simulink model "modelo_motor_P4_2"  (R2021b)
settings: Solver=VariableStepAuto  StartTime=0.0  StopTime=Tend  RelTol=1e-3
values from neighbouring files (symbols this model uses):
  Kd = Kp*Td    (= 0.01)    [lanza_P4_2.m]
  Ki = Kp/Ti    (= 8.33333333333)    [lanza_P4_2.m]
  Kp = 5    [lanza_P4_2.m]
  Td = 0.002    [lanza_P4_2.m]
  Ti = 0.6    [lanza_P4_2.m]
  Tm = 0.01    [lanza_P4_1.m]    (also in lanza_P4_2.m)
undefined symbols (not defined in the file or in its folder): k_bc, V_sat
libraries: cstblocks x6, slpidlib x1, dspsrcs4 x1
settings Model: Creator=jvalls  LastModifiedBy=jgragia
settings SolverCC: AlgebraicLoopSolver=TrustRegion
settings DataIOCC: ReturnWorkspaceOutputs=off
settings DebuggingCC: SFMachineParentedDataDiag=warning  ArithmeticOperatorsInVariantConditions=warning
settings SFSimCC: SimUseLocalCustomCode=off  CustomCodeUndefinedFunction=UseInterfaceOnly
settings RTWCC: RTWUseLocalCustomCode=off

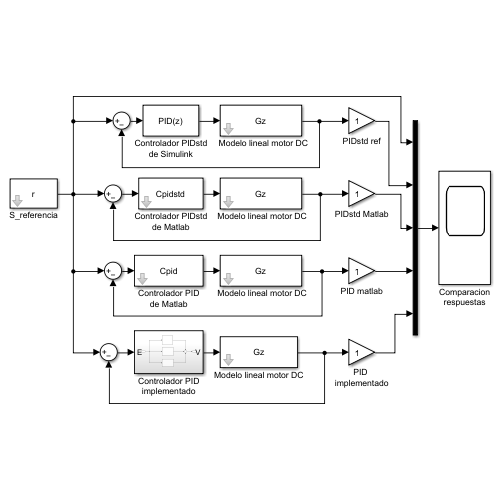
[thumbnail: Simulink's stored preview of the top-level diagram]
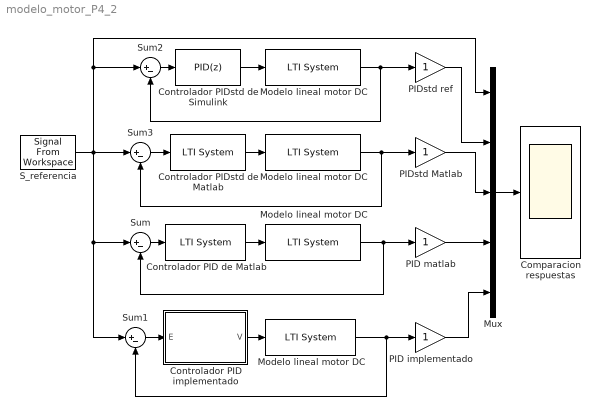
== system modelo_motor_P4_2 ==
  "       Modelo lineal motor DC      " : cstblocks/LTI System  sys=Gz  IC=[]
  "     Modelo lineal motor DC    " : cstblocks/LTI System  sys=Gz  IC=[]
  "    Modelo lineal motor DC  " : cstblocks/LTI System  sys=Gz  IC=[]
  "  Modelo lineal motor DC  " : cstblocks/LTI System  sys=Gz  IC=[]
  Comparacion respuestas : Scope
  Controlador PID de Matlab : cstblocks/LTI System  sys=Cpid  IC=[]
  Controlador PID implementado : Subsystem
  Controlador PIDstd de Matlab : cstblocks/LTI System  sys=Cpidstd  IC=[]
  Controlador PIDstd de Simulink : slpidlib/PID Controller  Controller=PID  Form=Ideal  TimeDomain=Discrete-time  UseExternalTs=off  SampleTime=Tm  IntegratorMethod=Backward Euler  FilterMethod=Forward Euler  ControllerParametersSource=internal  P=Kp  I=1/Ti  D=Td  UseFilter=off  N=100  TunerSelectOption=Transfer Function Based (PID Tuner App)  ZeroCross=off  InitialConditionSource=internal  InitialConditionForIntegrator=0  InitialConditionForFilter=0  DifferentiatorICPrevScaledInput=0  ExternalReset=none  TrackingMode=off  Kt=1  LimitOutput=off  SatLimitsSource=internal  UpperSaturationLimit=V_sat  LowerSaturationLimit=-V_sat  LinearizeAsGain=off  AntiWindupMode=back-calculation  Kb=k_bc  POutMin=[]  POutMax=[]  IOutMin=[]  IOutMax=[]  DOutMin=[]  DOutMax=[]  NOutMin=[]  NOutMax=[]  SumOutMin=[]  SumOutMax=[]  SaturationOutMin=[]  SaturationOutMax=[]  PParamMin=[]  PParamMax=[]  IParamMin=[]  IParamMax=[]  DParamMin=[]  DParamMax=[]  NParamMin=[]  NParamMax=[]  KbParamMin=[]  KbParamMax=[]  KtParamMin=[]  KtParamMax=[]  KbOutMin=[]  KbOutMax=[]  KtOutMin=[]  KtOutMax=[]  IntegratorOutMin=[]  IntegratorOutMax=[]  FilterOutMin=[]  FilterOutMax=[]  SumI1OutMin=[]  SumI1OutMax=[]  SumI2OutMin=[]  SumI2OutMax=[]  SumI3OutMin=[]  SumI3OutMax=[]  SumI4OutMin=[]  SumI4OutMax=[]  SumDOutMin=[]  SumDOutMax=[]  DifferentiatorOutMin=[]  DifferentiatorOutMax=[]  FilterDiffOutCoefMin=[]  FilterDiffOutCoefMax=[]  ReciprocalOutMin=[]  ReciprocalOutMax=[]  SumDenOutMin=[]  SumDenOutMax=[]  SumNumOutMin=[]  SumNumOutMax=[]  DivideOutMin=[]  DivideOutMax=[]  UdiffTsProdOutMin=[]  UdiffTsProdOutMax=[]  NTsProdOutMin=[]  NTsProdOutMax=[]  UintegralTsProdOutMin=[]  UintegralTsProdOutMax=[]  UngainTsProdOutMin=[]  UngainTsProdOutMax=[]  IntegratorContinuousStateAttributes=''  IntegratorStateMustResolveToSignalObject=off  IntegratorRTWStateStorageClass=Auto  FilterContinuousStateAttributes=''  FilterStateMustResolveToSignalObject=off  FilterRTWStateStorageClass=Auto  ParallelPVariant=Passthrough  IdealPVariant=InternalParameters  IVariant=InternalParameters  DVariant=InternalParameters  IntegratorVariant=Discrete  SatVariant=Disabled  AWVariant=Passthrough  PCopyVariant=Disabled  TRVariant=Disabled  FdbkBlocksVariant=Forward  IdealPFdbkVariant=Disabled  SatFdbkVariant=Disabled  DerivativeFilterVariant=Differentiator  NVariant=Passthrough  NCopyVariant=Disabled_SignalSpec  FilterICVariant=InternalICsDifferentiator  IntegratorICVariant=InternalICs  ExternalResetVariant=Disabled  TRSumVariant=Passthrough  SumFdbkVariant=Disabled  SumVariant=Sum_PID  TsampFilterVariant=InternalTs  TsampNgainVariant=Passthrough  TsampIntegralVariant=Passthrough  ExternalSaturationOutDataTypeStr=Inherit: Same as second input
  Mux : Mux  Inputs=5
  PID implementado : Gain
  PID matlab : Gain
  PIDstd Matlab : Gain
  PIDstd ref : Gain
  S_referencia : dspsrcs4/Signal From Workspace  X=r  Ts=Tm  nsamps=1  OutputAfterFinalValue=Setting to zero  ignoreOrWarnInputAndFrameLengths=off  OutputFrames=off
  Sum{,1..3} (4 alike) : Sum  Inputs=|+-
  wires:
  Mux/1 -> Comparacion respuestas/1
  Sum/1 -> Controlador PID de Matlab/1
  Controlador PID implementado/1(V) -> "  Modelo lineal motor DC  "/1
  "     Modelo lineal motor DC    "/1 -> PID matlab/1, Sum/2
  Controlador PID de Matlab/1 -> "     Modelo lineal motor DC    "/1
  "  Modelo lineal motor DC  "/1 -> PID implementado/1, Sum1/2
  Sum1/1 -> Controlador PID implementado/1(E)
  Controlador PIDstd de Simulink/1 -> "    Modelo lineal motor DC  "/1
  Sum2/1 -> Controlador PIDstd de Simulink/1
  "    Modelo lineal motor DC  "/1 -> PIDstd ref/1, Sum2/2
  Controlador PIDstd de Matlab/1 -> "       Modelo lineal motor DC      "/1
  "       Modelo lineal motor DC      "/1 -> PIDstd Matlab/1, Sum3/2
  Sum3/1 -> Controlador PIDstd de Matlab/1
  S_referencia/1 -> Mux/1, Sum2/1, Sum3/1, Sum1/1, Sum/1
  PIDstd ref/1 -> Mux/2
  PIDstd Matlab/1 -> Mux/3
  PID matlab/1 -> Mux/4
  PID implementado/1 -> Mux/5

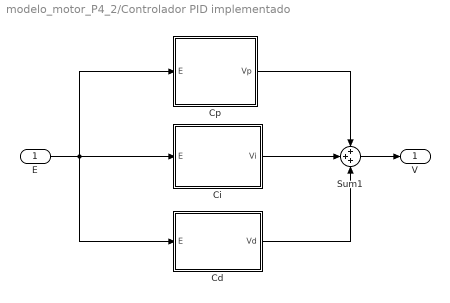
== system modelo_motor_P4_2/Controlador PID implementado ==
  E : Inport
  Cd : Subsystem
  Ci : Subsystem
  Cp : Subsystem
  Sum1 : Sum  Inputs=+++
  V : Outport  VectorParamsAs1DForOutWhenUnconnected=off
  wires:
  Sum1/1 -> V/1
  Cp/1(Vp) -> Sum1/1
  Ci/1(Vi) -> Sum1/2
  Cd/1(Vd) -> Sum1/3
  E/1 -> Cd/1(E), Cp/1(E), Ci/1(E)

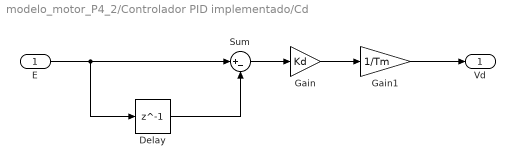
== system modelo_motor_P4_2/Controlador PID implementado/Cd ==
  E : Inport
  Delay : Delay  DelayLength=1  InitialCondition=0
  Gain : Gain  Gain=Kd
  Gain1 : Gain  Gain=1/Tm
  Sum : Sum  Inputs=|+-
  Vd : Outport  VectorParamsAs1DForOutWhenUnconnected=off
  wires:
  Gain/1 -> Gain1/1
  Gain1/1 -> Vd/1
  Sum/1 -> Gain/1
  E/1 -> Delay/1, Sum/1
  Delay/1 -> Sum/2

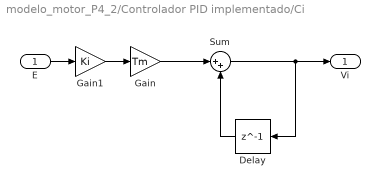
== system modelo_motor_P4_2/Controlador PID implementado/Ci ==
  E : Inport
  Delay : Delay  DelayLength=1  InitialCondition=0
  Gain : Gain  Gain=Tm
  Gain1 : Gain  Gain=Ki
  Sum : Sum  Inputs=|++
  Vi : Outport  VectorParamsAs1DForOutWhenUnconnected=off
  wires:
  E/1 -> Gain1/1
  Gain1/1 -> Gain/1
  Gain/1 -> Sum/1
  Sum/1 -> Delay/1, Vi/1
  Delay/1 -> Sum/2

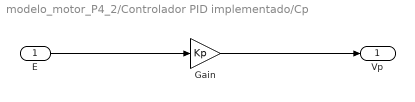
== system modelo_motor_P4_2/Controlador PID implementado/Cp ==
  E : Inport
  Gain : Gain  Gain=Kp
  Vp : Outport  VectorParamsAs1DForOutWhenUnconnected=off
  wires:
  E/1 -> Gain/1
  Gain/1 -> Vp/1
